simulink model "testemplanner_cs"  (R2023a)
settings: Solver=ode5  StartTime=0.0  StopTime=60  FixedStep=1/1000  RelTol=1e-3
PreLoadFcn:
  | mbxruntime.callbacks.PreLoadFcn(bdroot);
PostLoadFcn:
  | mbxruntime.callbacks.PostLoadFcn(bdroot);
InitFcn:
  | mbxruntime.callbacks.InitFcn(bdroot);
StartFcn:
  | mbxruntime.callbacks.StartFcn(bdroot);
StopFcn:
  | mbxruntime.callbacks.StopFcn(bdroot);
model workspace (MAT data in the model file):
  mbox_table : object (value not decoded)
  model_closed = 0
  sim_status = 0
undefined symbols (not defined in the file): aubr, c_factor, cf, cr, DiscIntNeverNeededParam, global_path_x, global_path_y, KD_PID_distance, KD_PID_speed, KI_PID_distance, KI_PID_speed, KP_PID_distance, KP_PID_speed, la, lb, LQR_K1, LQR_K2, LQR_K3, LQR_K4, m, rack_displacement, right_wheel_ground, tablebr, vubr, vx_break_point
libraries: PreScanSimulinkLibrary x14, Solver_SF x1
(part 5 of 8)

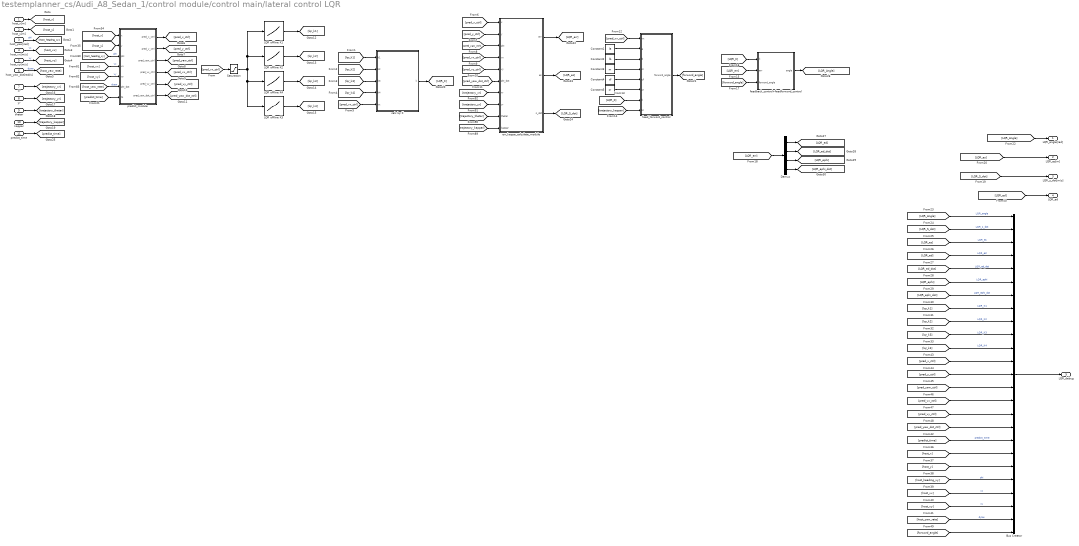
== system testemplanner_cs/Audi_A8_Sedan_1/control module/control main/lateral control LQR ==
  host_x[m] : Inport
  host_y[m] : Inport  Port=2
  host_yaw[rad] : Inport  Port=3
  host_vx[m/s] : Inport  Port=4
  host_vy[m/s] : Inport  Port=5
  host_yaw_dot[rad/s] : Inport  Port=6
  xr : Inport  Port=7
  yr : Inport  Port=8
  thetar : Inport  Port=9
  kappar : Inport  Port=10
  predict_time : Inport  Port=11
  Bus Creator : BusCreator  Inputs=25
  Constant1 : Constant  Value=la
  Constant2 : Constant  Value=lb
  Constant3 : Constant  Value=m
  Constant4 : Constant  Value=cf
  Constant5 : Constant  Value=cr
  Demux : Demux
  LQR offline K1 : Lookup_n-D  NumberOfTableDimensions=1  BreakpointsForDimension1=vx_break_point  Table=LQR_K1  InternalRulePriority=Speed  RndMeth=Simplest
  LQR offline K2 : Lookup_n-D  NumberOfTableDimensions=1  BreakpointsForDimension1=vx_break_point  Table=LQR_K2  InternalRulePriority=Speed  RndMeth=Simplest
  LQR offline K3 : Lookup_n-D  NumberOfTableDimensions=1  BreakpointsForDimension1=vx_break_point  Table=LQR_K3  InternalRulePriority=Speed  RndMeth=Simplest
  LQR offline K4 : Lookup_n-D  NumberOfTableDimensions=1  BreakpointsForDimension1=vx_break_point  Table=LQR_K4  InternalRulePriority=Speed  RndMeth=Simplest
  Saturation : Saturate  UpperLimit=50  LowerLimit=0
  calc lqr K : MATLAB Function  TreatAsAtomicUnit=on
  err_kappa_calculate_module : MATLAB Function  TreatAsAtomicUnit=on
  feed_forword_control : MATLAB Function  TreatAsAtomicUnit=on
  feedback_control+feedforword_control : MATLAB Function  TreatAsAtomicUnit=on
  predict_module : MATLAB Function  TreatAsAtomicUnit=on
  LQR_angle[rad] : Outport  VectorParamsAs1DForOutWhenUnconnected=off
  LQR_es[m] : Outport  Port=2  VectorParamsAs1DForOutWhenUnconnected=off
  LQR_s_dot[m/s] : Outport  Port=3  VectorParamsAs1DForOutWhenUnconnected=off
  LQR_ed : Outport  Port=4  VectorParamsAs1DForOutWhenUnconnected=off
  LQR_debug : Outport  Port=5  VectorParamsAs1DForOutWhenUnconnected=off
  wires:
  [host_vy] -> predict_module/5(vy)  "vy"
  [host_x] -> predict_module/1(x)
  [host_yaw_rate] -> predict_module/6(phi_dot)  "dyaw"
  [host_vx] -> predict_module/4(vx)  "vx"
  [host_y] -> predict_module/2(y)
  [host_heading_xy] -> predict_module/3(phi)  "phi"
  [predict_time] -> predict_module/7(ts)
  host_x[m]/1 -> [host_x]
  host_y[m]/1 -> [host_y]
  host_yaw[rad]/1 -> [host_heading_xy]  "phi"
  host_vx[m/s]/1 -> [host_vx]  "vx"
  host_vy[m/s]/1 -> [host_vy]  "vy"
  host_yaw_dot[rad/s]/1 -> [host_yaw_rate]  "dyaw"
  predict_module/1(pred_x_ctrl) -> [pred_x_ctrl]
  predict_module/2(pred_y_ctrl) -> [pred_y_ctrl]
  predict_module/3(pred_yaw_ctrl) -> [pred_yaw_ctrl]
  predict_module/4(pred_vx_ctrl) -> [pred_vx_ctrl]
  predict_module/5(pred_vy_ctrl) -> [pred_vy_ctrl]
  predict_module/6(pred_yaw_dot_ctrl) -> [pred_yaw_dot_ctrl]
  [pred_vx_ctrl] -> Saturation/1
  LQR offline K1/1 -> [lqr_k1]
  LQR offline K2/1 -> [lqr_k2]
  LQR offline K4/1 -> [lqr_k3]
  LQR offline K3/1 -> [lqr_k4]
  [pred_vx_ctrl] -> calc lqr K/5(vx)
  [lqr_k4] -> calc lqr K/4(k4)
  [lqr_k3] -> calc lqr K/3(k3)
  [lqr_k2] -> calc lqr K/2(k2)
  [lqr_k1] -> calc lqr K/1(k1)
  [pred_x_ctrl] -> err_kappa_calculate_module/1(x)
  [pred_y_ctrl] -> err_kappa_calculate_module/2(y)
  [pred_yaw_ctrl] -> err_kappa_calculate_module/3(phi)
  [pred_vx_ctrl] -> err_kappa_calculate_module/4(vx)
  [pred_vy_ctrl] -> err_kappa_calculate_module/5(vy)
  [pred_yaw_dot_ctrl] -> err_kappa_calculate_module/6(phi_dot)
  xr/1 -> [trajectory_xr]
  yr/1 -> [trajectory_yr]
  thetar/1 -> [trajectory_thetar]
  kappar/1 -> [trajectory_kappar]
  [trajectory_xr] -> err_kappa_calculate_module/7(xr)
  [trajectory_yr] -> err_kappa_calculate_module/8(yr)
  [trajectory_kappar] -> err_kappa_calculate_module/10(kappar)
  [trajectory_thetar] -> err_kappa_calculate_module/9(thetar)
  [pred_vx_ctrl] -> feed_forword_control/1(vx)
  Constant1/1 -> feed_forword_control/2(a)
  Constant2/1 -> feed_forword_control/3(b)
  Constant3/1 -> feed_forword_control/4(m)
  Constant4/1 -> feed_forword_control/5(cf)
  Constant5/1 -> feed_forword_control/6(cr)
  calc lqr K/1(k) -> [LQR_K]
  [LQR_K] -> feed_forword_control/7(k)
  [trajectory_kappar] -> feed_forword_control/8(kr)
  feed_forword_control/1(forword_angle) -> [forword_angle]
  err_kappa_calculate_module/1(err) -> [LQR_err]
  [LQR_err] -> feedback_control+feedforword_control/2(err)
  [LQR_K] -> feedback_control+feedforword_control/1(k)
  [forword_angle] -> feedback_control+feedforword_control/3(forword_angle)
  [LQR_err] -> Demux/1
  err_kappa_calculate_module/2(es) -> [LQR_es]
  err_kappa_calculate_module/3(s_dot) -> [LQR_S_dot]
  [LQR_S_dot] -> LQR_s_dot[m/s]/1
  [LQR_es] -> LQR_es[m]/1
  Saturation/1 -> LQR offline K3/1, LQR offline K4/1, LQR offline K2/1, LQR offline K1/1
  predict_time/1 -> [predict_time]
  Bus Creator/1 -> LQR_debug/1
  feedback_control+feedforword_control/1(angle) -> [LQR_Angle]
  [LQR_Angle] -> LQR_angle[rad]/1
  [LQR_Angle] -> Bus Creator/1  "LQR_angle"
  [LQR_S_dot] -> Bus Creator/2  "LQR_s_dot"
  [LQR_es] -> Bus Creator/3  "LQR_es"
  Demux/1 -> [LQR_ed]
  Demux/2 -> [LQR_ed_dot]
  Demux/3 -> [LQR_ephi]
  Demux/4 -> [LQR_ephi_dot]
  [LQR_ed] -> Bus Creator/4  "LQR_ed"
  [LQR_ed_dot] -> Bus Creator/5  "LQR_ed_dot"
  [LQR_ephi] -> Bus Creator/6  "LQR_ephi"
  [LQR_ephi_dot] -> Bus Creator/7  "LQR_ephi_dot"
  [lqr_k1] -> Bus Creator/8  "LQR_K1"
  [lqr_k2] -> Bus Creator/9  "LQR_K2"
  [lqr_k3] -> Bus Creator/10  "LQR_K3"
  [lqr_k4] -> Bus Creator/11  "LQR_K4"
  [pred_x_ctrl] -> Bus Creator/12
  [pred_y_ctrl] -> Bus Creator/13
  [pred_yaw_ctrl] -> Bus Creator/14
  [pred_vx_ctrl] -> Bus Creator/15
  [pred_vy_ctrl] -> Bus Creator/16
  [pred_yaw_dot_ctrl] -> Bus Creator/17
  [predict_time] -> Bus Creator/18  "predict_time"
  [host_x] -> Bus Creator/19
  [host_y] -> Bus Creator/20
  [host_heading_xy] -> Bus Creator/21  "phi"
  [host_vx] -> Bus Creator/22  "vx"
  [host_vy] -> Bus Creator/23  "vy"
  [host_yaw_rate] -> Bus Creator/24  "dyaw"
  [forword_angle] -> Bus Creator/25
  [LQR_ed] -> LQR_ed/1

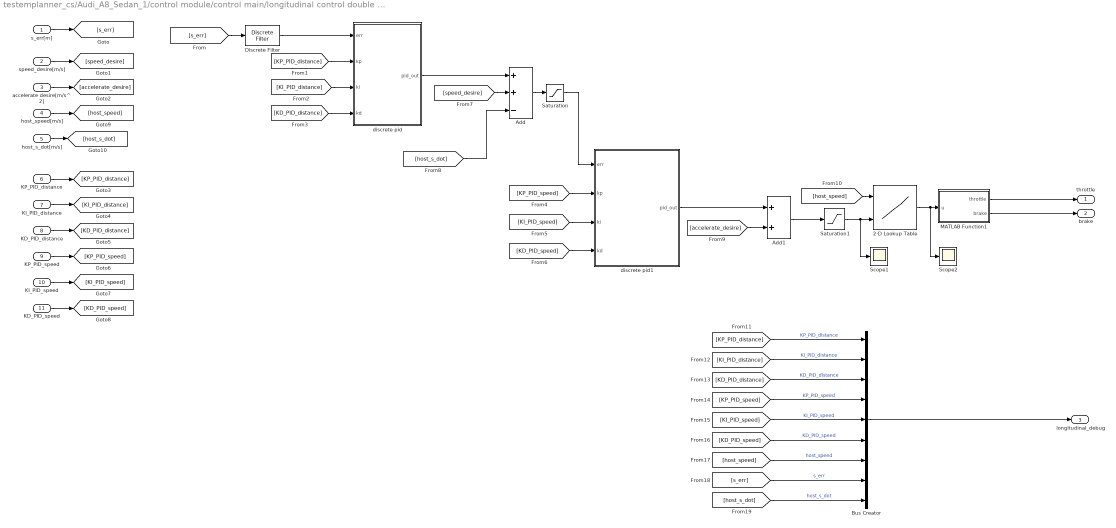
== system testemplanner_cs/Audi_A8_Sedan_1/control module/control main/longitudinal control double PID ==
  s_err[m] : Inport
  speed_desire[m/s] : Inport  Port=2
  accelerate desire[m/s^2] : Inport  Port=3
  host_speed[m/s] : Inport  Port=4
  host_s_dot[m/s] : Inport  Port=5
  KP_PID_distance : Inport  Port=6
  KI_PID_distance : Inport  Port=7
  KD_PID_distance : Inport  Port=8
  KP_PID_speed : Inport  Port=9
  KI_PID_speed : Inport  Port=10
  KD_PID_speed : Inport  Port=11
  2-D Lookup Table : Lookup_n-D  BreakpointsForDimension1=vubr  BreakpointsForDimension2=aubr  Table=tablebr  InternalRulePriority=Speed  RndMeth=Simplest
      settings: InputPortMap=u0,u1
  Add : Sum  Inputs=++-
  Add1 : Sum
  Bus Creator : BusCreator  Inputs=9
  Discrete Filter : DiscreteFilter
  MATLAB Function1 : MATLAB Function  TreatAsAtomicUnit=on
  Saturation : Saturate  UpperLimit=45  LowerLimit=-45
  Saturation1 : Saturate  UpperLimit=5  LowerLimit=-8
  Scope1 : Scope
  Scope2 : Scope
  discrete pid : Subsystem
  discrete pid1 : Subsystem
  throttle : Outport
  brake : Outport  Port=2
  longitudinal_debug : Outport  Port=3
  wires:
  2-D Lookup Table/1 -> Scope2/1, MATLAB Function1/1(u)
  s_err[m]/1 -> [s_err]
  speed_desire[m/s]/1 -> [speed_desire]
  accelerate desire[m/s^2]/1 -> [accelerate_desire]
  KP_PID_distance/1 -> [KP_PID_distance]
  KI_PID_distance/1 -> [KI_PID_distance]
  KD_PID_distance/1 -> [KD_PID_distance]
  KP_PID_speed/1 -> [KP_PID_speed]
  KI_PID_speed/1 -> [KI_PID_speed]
  KD_PID_speed/1 -> [KD_PID_speed]
  [s_err] -> Discrete Filter/1
  [KP_PID_distance] -> discrete pid/2(kp)
  [KI_PID_distance] -> discrete pid/3(ki)
  [KD_PID_distance] -> discrete pid/4(kd)
  [KP_PID_speed] -> discrete pid1/2(kp)
  [KI_PID_speed] -> discrete pid1/3(ki)
  [KD_PID_speed] -> discrete pid1/4(kd)
  host_speed[m/s]/1 -> [host_speed]
  discrete pid/1(pid_out) -> Add/1
  [speed_desire] -> Add/2
  Add/1 -> Saturation/1
  Saturation/1 -> discrete pid1/1(err)
  discrete pid1/1(pid_out) -> Add1/1
  [accelerate_desire] -> Add1/2
  Add1/1 -> Saturation1/1
  Saturation1/1 -> Scope1/1, 2-D Lookup Table/2
  host_s_dot[m/s]/1 -> [host_s_dot]
  [host_s_dot] -> Add/3
  [host_speed] -> 2-D Lookup Table/1
  Discrete Filter/1 -> discrete pid/1(err)
  MATLAB Function1/1(throttle) -> throttle/1
  MATLAB Function1/2(brake) -> brake/1
  [KP_PID_distance] -> Bus Creator/1  "KP_PID_distance"
  [KI_PID_distance] -> Bus Creator/2  "KI_PID_distance"
  [KD_PID_distance] -> Bus Creator/3  "KD_PID_distance"
  [KP_PID_speed] -> Bus Creator/4  "KP_PID_speed"
  [KI_PID_speed] -> Bus Creator/5  "KI_PID_speed"
  [KD_PID_speed] -> Bus Creator/6  "KD_PID_speed"
  [host_speed] -> Bus Creator/7  "host_speed"
  [s_err] -> Bus Creator/8  "s_err"
  [host_s_dot] -> Bus Creator/9  "host_s_dot"
  Bus Creator/1 -> longitudinal_debug/1

== system testemplanner_cs/Audi_A8_Sedan_1/control module/control main/understeer compensate ==
  LQR_angle : Inport
  lateral err : Inport  Port=2
  Add : Sum  Inputs=+-
  Gain : Gain  Gain=0.01
  Manual Switch : ManualSwitch
  LQR_final_angle : Outport
  wires:
  Add/1 -> Manual Switch/2
  Gain/1 -> Add/2
  lateral err/1 -> Gain/1
  LQR_angle/1 -> Add/1, Manual Switch/1
  Manual Switch/1 -> LQR_final_angle/1

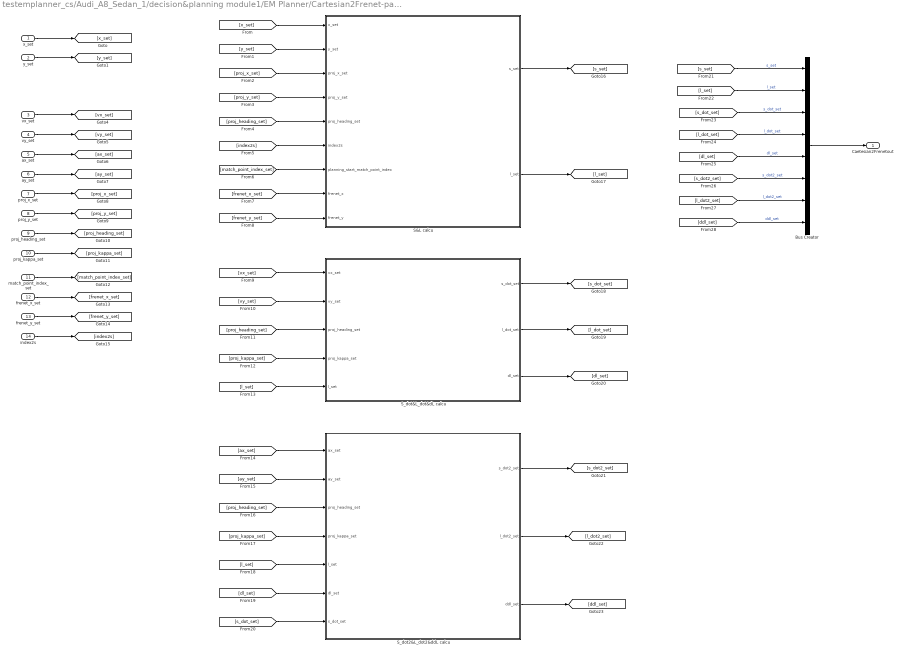
== system testemplanner_cs/Audi_A8_Sedan_1/decision&planning module1/EM Planner/Cartesian2Frenet-panning start point ==
  x_set : Inport
  y_set : Inport  Port=2
  vx_set : Inport  Port=3
  vy_set : Inport  Port=4
  ax_set : Inport  Port=5
  ay_set : Inport  Port=6
  proj_x_set : Inport  Port=7
  proj_y_set : Inport  Port=8
  proj_heading_set : Inport  Port=9
  proj_kappa_set : Inport  Port=10
  match_point_index_set : Inport  Port=11
  frenet_x_set : Inport  Port=12
  frenet_y_set : Inport  Port=13
  index2s : Inport  Port=14
  Bus Creator : BusCreator  Inputs=8
  S&L calcu : MATLAB Function  TreatAsAtomicUnit=on
  "S_dot&L_dot&dL calcu " : MATLAB Function  TreatAsAtomicUnit=on
  S_dot2&L_dot2&ddL calcu : MATLAB Function  TreatAsAtomicUnit=on
  Caetesian2Frenetout : Outport
  wires:
  x_set/1 -> [x_set]
  y_set/1 -> [y_set]
  vx_set/1 -> [vx_set]
  vy_set/1 -> [vy_set]
  ax_set/1 -> [ax_set]
  ay_set/1 -> [ay_set]
  proj_x_set/1 -> [proj_x_set]
  proj_y_set/1 -> [proj_y_set]
  proj_heading_set/1 -> [proj_heading_set]
  proj_kappa_set/1 -> [proj_kappa_set]
  match_point_index_set/1 -> [match_point_index_set]
  frenet_x_set/1 -> [frenet_x_set]
  frenet_y_set/1 -> [frenet_y_set]
  index2s/1 -> [index2s]
  [y_set] -> S&L calcu/2(y_set)
  [proj_x_set] -> S&L calcu/3(proj_x_set)
  [proj_y_set] -> S&L calcu/4(proj_y_set)
  [x_set] -> S&L calcu/1(x_set)
  [proj_heading_set] -> S&L calcu/5(proj_heading_set)
  [index2s] -> S&L calcu/6(index2s)
  [match_point_index_set] -> S&L calcu/7(planning_start_match_point_index)
  [frenet_x_set] -> S&L calcu/8(frenet_x)
  [frenet_y_set] -> S&L calcu/9(frenet_y)
  [vx_set] -> "S_dot&L_dot&dL calcu "/1(vx_set)
  [vy_set] -> "S_dot&L_dot&dL calcu "/2(vy_set)
  [proj_heading_set] -> "S_dot&L_dot&dL calcu "/3(proj_heading_set)
  [proj_kappa_set] -> "S_dot&L_dot&dL calcu "/4(proj_kappa_set)
  S&L calcu/1(s_set) -> [s_set]
  S&L calcu/2(l_set) -> [l_set]
  [l_set] -> "S_dot&L_dot&dL calcu "/5(l_set)
  "S_dot&L_dot&dL calcu "/1(s_dot_set) -> [s_dot_set]
  "S_dot&L_dot&dL calcu "/2(l_dot_set) -> [l_dot_set]
  "S_dot&L_dot&dL calcu "/3(dl_set) -> [dl_set]
  [ax_set] -> S_dot2&L_dot2&ddL calcu/1(ax_set)
  [ay_set] -> S_dot2&L_dot2&ddL calcu/2(ay_set)
  [proj_heading_set] -> S_dot2&L_dot2&ddL calcu/3(proj_heading_set)
  [proj_kappa_set] -> S_dot2&L_dot2&ddL calcu/4(proj_kappa_set)
  [l_set] -> S_dot2&L_dot2&ddL calcu/5(l_set)
  [dl_set] -> S_dot2&L_dot2&ddL calcu/6(dl_set)
  [s_dot_set] -> S_dot2&L_dot2&ddL calcu/7(s_dot_set)
  S_dot2&L_dot2&ddL calcu/1(s_dot2_set) -> [s_dot2_set]
  S_dot2&L_dot2&ddL calcu/2(l_dot2_set) -> [l_dot2_set]
  S_dot2&L_dot2&ddL calcu/3(ddl_set) -> [ddl_set]
  [s_set] -> Bus Creator/1  "s_set"
  [l_set] -> Bus Creator/2  "l_set"
  [s_dot_set] -> Bus Creator/3  "s_dot_set"
  [l_dot_set] -> Bus Creator/4  "l_dot_set"
  [dl_set] -> Bus Creator/5  "dl_set"
  [s_dot2_set] -> Bus Creator/6  "s_dot2_set"
  [l_dot2_set] -> Bus Creator/7  "l_dot2_set"
  [ddl_set] -> Bus Creator/8  "ddl_set"
  Bus Creator/1 -> Caetesian2Frenetout/1

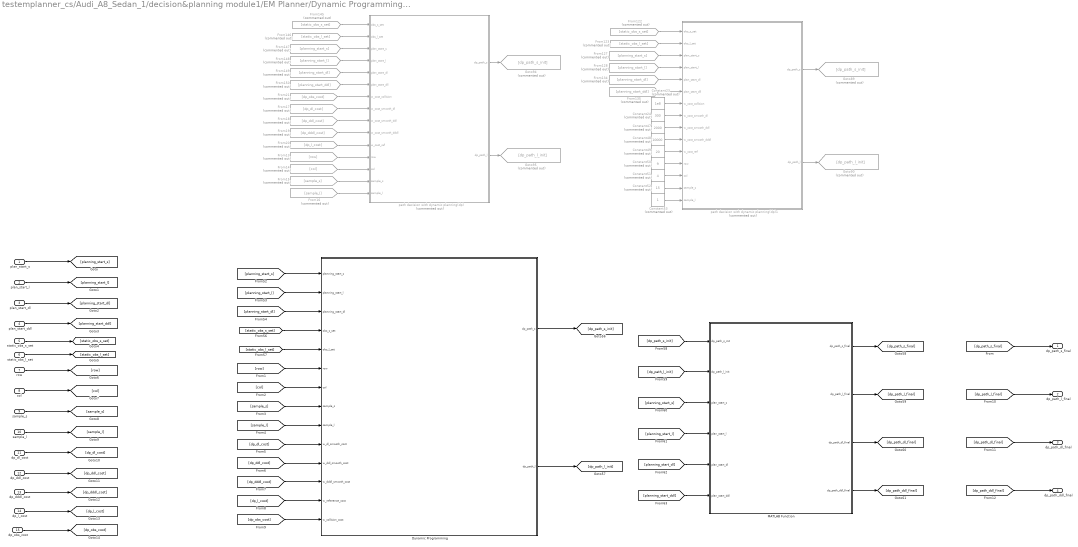
== system testemplanner_cs/Audi_A8_Sedan_1/decision&planning module1/EM Planner/Dynamic Programming&Increase DP Node ==
  plan_start_s : Inport
  plan_start_l : Inport  Port=2
  plan_start_dl : Inport  Port=3
  plan_start_ddl : Inport  Port=4
  static_obs_s_set : Inport  Port=5
  static_obs_l_set : Inport  Port=6
  row : Inport  Port=7
  col : Inport  Port=8
  sample_s : Inport  Port=9
  sample_l : Inport  Port=10
  dp_dl_cost : Inport  Port=11
  dp_ddl_cost : Inport  Port=12
  dp_dddl_cost : Inport  Port=13
  dp_l_cost : Inport  Port=14
  dp_obs_cost : Inport  Port=15
  Constant23 : Constant  Commented=on  Value=1e8
  Constant24 : Constant  Commented=on  Value=300
  Constant47 : Constant  Commented=on  Value=2000
  Constant48 : Constant  Commented=on  Value=10000
  Constant49 : Constant  Commented=on  Value=20
  Constant50 : Constant  Commented=on  Value=9
  Constant51 : Constant  Commented=on  Value=4
  Constant52 : Constant  Commented=on  Value=15
  Constant53 : Constant  Commented=on
  Dynamic Programming : MATLAB Function  TreatAsAtomicUnit=on
  From122 : From  Commented=on  GotoTag=static_obs_s_set
  From123 : From  Commented=on  GotoTag=static_obs_l_set
  From127 : From  Commented=on  GotoTag=planning_start_s
  From128 : From  Commented=on  GotoTag=planning_start_l
  From13 : From  Commented=on  GotoTag=row
  From134 : From  Commented=on  GotoTag=planning_start_dl
  From135 : From  Commented=on  GotoTag=planning_start_ddl
  From14 : From  Commented=on  GotoTag=col
  From145 : From  Commented=on  GotoTag=static_obs_s_set
  From146 : From  Commented=on  GotoTag=static_obs_l_set
  From147 : From  Commented=on  GotoTag=planning_start_s
  From148 : From  Commented=on  GotoTag=planning_start_l
  From149 : From  Commented=on  GotoTag=planning_start_dl
  From15 : From  Commented=on  GotoTag=sample_s
  From150 : From  Commented=on  GotoTag=planning_start_ddl
  From16 : From  Commented=on  GotoTag=sample_l
  From17 : From  Commented=on  GotoTag=dp_dl_cost
  From18 : From  Commented=on  GotoTag=dp_ddl_cost
  From19 : From  Commented=on  GotoTag=dp_dddl_cost
  From20 : From  Commented=on  GotoTag=dp_l_cost
  From21 : From  Commented=on  GotoTag=dp_obs_cost
  Goto89 : Goto  Commented=on  GotoTag=dp_path_s_init
  Goto90 : Goto  Commented=on  GotoTag=dp_path_l_init
  Goto94 : Goto  Commented=on  GotoTag=dp_path_s_init
  Goto95 : Goto  Commented=on  GotoTag=dp_path_l_init
  MATLAB Function : MATLAB Function  TreatAsAtomicUnit=on
  path decision with dynamic planning(dp) : MATLAB Function  Commented=on  TreatAsAtomicUnit=on
  path decision with dynamic planning(dp)1 : MATLAB Function  Commented=on  TreatAsAtomicUnit=on
  dp_path_s_final : Outport
  dp_path_l_final : Outport  Port=2
  dp_path_dl_final : Outport  Port=3
  dp_path_ddl_final : Outport  Port=4
  wires:
  Constant23/1 -> path decision with dynamic planning(dp)1/7(w_cost_collision)
  From21/1 -> path decision with dynamic planning(dp)/7(w_cost_collision)
  Constant47/1 -> path decision with dynamic planning(dp)1/9(w_cost_smooth_ddl)
  Constant49/1 -> path decision with dynamic planning(dp)1/11(w_cost_ref)
  Constant24/1 -> path decision with dynamic planning(dp)1/8(w_cost_smooth_dl)
  [row] -> Dynamic Programming/6(row)
  [sample_s] -> Dynamic Programming/8(sample_s)
  From19/1 -> path decision with dynamic planning(dp)/10(w_cost_smooth_dddl)
  Constant50/1 -> path decision with dynamic planning(dp)1/12(row)
  MATLAB Function/3(dp_path_dl_final) -> [dp_path_dl_final]
  [col] -> Dynamic Programming/7(col)
  MATLAB Function/1(dp_path_s_final) -> [dp_path_s_final]
  Constant48/1 -> path decision with dynamic planning(dp)1/10(w_cost_smooth_dddl)
  From128/1 -> path decision with dynamic planning(dp)1/4(plan_start_l)
  From123/1 -> path decision with dynamic planning(dp)1/2(obs_l_set)
  From134/1 -> path decision with dynamic planning(dp)1/5(plan_start_dl)
  path decision with dynamic planning(dp)/2(dp_path_l) -> Goto95/1
  path decision with dynamic planning(dp)1/1(dp_path_s) -> Goto89/1
  [planning_start_l] -> MATLAB Function/4(plan_start_l)
  [planning_start_dl] -> Dynamic Programming/3(planning_start_dl)
  From17/1 -> path decision with dynamic planning(dp)/8(w_cost_smooth_dl)
  From16/1 -> path decision with dynamic planning(dp)/15(sample_l)
  path decision with dynamic planning(dp)1/2(dp_path_l) -> Goto90/1
  Constant52/1 -> path decision with dynamic planning(dp)1/14(sample_s)
  Constant51/1 -> path decision with dynamic planning(dp)1/13(col)
  From135/1 -> path decision with dynamic planning(dp)1/6(plan_start_dll)
  From149/1 -> path decision with dynamic planning(dp)/5(plan_start_dl)
  From18/1 -> path decision with dynamic planning(dp)/9(w_cost_smooth_ddl)
  From122/1 -> path decision with dynamic planning(dp)1/1(obs_s_set)
  [dp_ddl_cost] -> Dynamic Programming/11(w_ddl_smooth_cost)
  Constant53/1 -> path decision with dynamic planning(dp)1/15(sample_l)
  [planning_start_l] -> Dynamic Programming/2(planning_start_l)
  From127/1 -> path decision with dynamic planning(dp)1/3(plan_start_s)
  [planning_start_s] -> MATLAB Function/3(plan_start_s)
  Dynamic Programming/1(dp_path_s) -> [dp_path_s_init]
  [dp_l_cost] -> Dynamic Programming/13(w_reference_cost)
  [static_obs_l_set] -> Dynamic Programming/5(obs_l_set)
  From15/1 -> path decision with dynamic planning(dp)/14(sample_s)
  From13/1 -> path decision with dynamic planning(dp)/12(row)
  [planning_start_s] -> Dynamic Programming/1(planning_start_s)
  From146/1 -> path decision with dynamic planning(dp)/2(obs_l_set)
  [dp_path_s_init] -> MATLAB Function/1(dp_path_s_init)
  [planning_start_ddl] -> MATLAB Function/6(plan_start_ddl)
  [static_obs_s_set] -> Dynamic Programming/4(obs_s_set)
  [dp_obs_cost] -> Dynamic Programming/14(w_collision_cost)
  [planning_start_dl] -> MATLAB Function/5(plan_start_dl)
  Dynamic Programming/2(dp_path_l) -> [dp_path_l_init]
  MATLAB Function/4(dp_path_ddl_final) -> [dp_path_ddl_final]
  [dp_path_l_init] -> MATLAB Function/2(dp_path_l_init)
  [dp_dl_cost] -> Dynamic Programming/10(w_dl_smooth_cost)
  [sample_l] -> Dynamic Programming/9(sample_l)
  MATLAB Function/2(dp_path_l_final) -> [dp_path_l_final]
  From14/1 -> path decision with dynamic planning(dp)/13(col)
  From145/1 -> path decision with dynamic planning(dp)/1(obs_s_set)
  path decision with dynamic planning(dp)/1(dp_path_s) -> Goto94/1
  From20/1 -> path decision with dynamic planning(dp)/11(w_cost_ref)
  From150/1 -> path decision with dynamic planning(dp)/6(plan_start_dll)
  From147/1 -> path decision with dynamic planning(dp)/3(plan_start_s)
  [dp_dddl_cost] -> Dynamic Programming/12(w_dddl_smooth_cost)
  From148/1 -> path decision with dynamic planning(dp)/4(plan_start_l)
  plan_start_s/1 -> [planning_start_s]
  plan_start_l/1 -> [planning_start_l]
  plan_start_dl/1 -> [planning_start_dl]
  plan_start_ddl/1 -> [planning_start_ddl]
  static_obs_s_set/1 -> [static_obs_s_set]
  static_obs_l_set/1 -> [static_obs_l_set]
  row/1 -> [row]
  col/1 -> [col]
  sample_s/1 -> [sample_s]
  sample_l/1 -> [sample_l]
  dp_dl_cost/1 -> [dp_dl_cost]
  dp_ddl_cost/1 -> [dp_ddl_cost]
  dp_dddl_cost/1 -> [dp_dddl_cost]
  dp_l_cost/1 -> [dp_l_cost]
  dp_obs_cost/1 -> [dp_obs_cost]
  [dp_path_s_final] -> dp_path_s_final/1
  [dp_path_l_final] -> dp_path_l_final/1
  [dp_path_dl_final] -> dp_path_dl_final/1
  [dp_path_ddl_final] -> dp_path_ddl_final/1

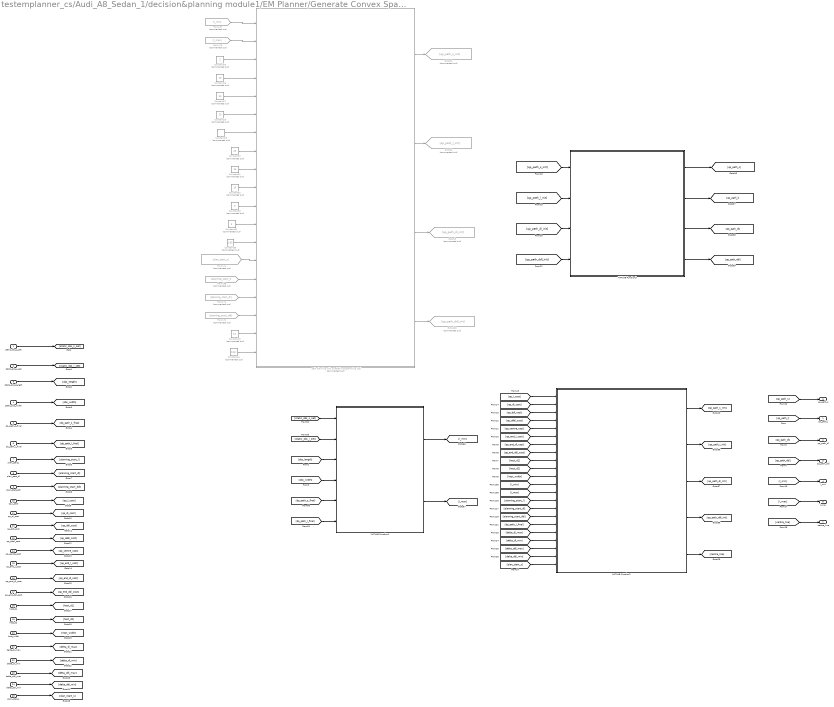
== system testemplanner_cs/Audi_A8_Sedan_1/decision&planning module1/EM Planner/Generate Convex Space&Quadratic Programming ==
  static_obs_s_set : Inport
  static_obs_l_set : Inport  Port=2
  static_obs_length : Inport  Port=3
  static_obs_width : Inport  Port=4
  dp_path_s_final : Inport  Port=5
  dp_path_l_final : Inport  Port=6
  plan_start_l : Inport  Port=7
  plan_start_dl : Inport  Port=8
  plan_start_ddl : Inport  Port=9
  qp_l_cost : Inport  Port=10
  qp_dl_cost : Inport  Port=11
  qp_ddl_cost : Inport  Port=12
  qp_dddl_cost : Inport  Port=13
  qp_centre_cost : Inport  Port=14
  qp_end_l_cost : Inport  Port=15
  qp_end_dl_cost : Inport  Port=16
  qp_end_ddl_cost : Inport  Port=17
  host_d1 : Inport  Port=18
  host_d2 : Inport  Port=19
  host_width : Inport  Port=20
  delta_dl_max : Inport  Port=21
  delta_dl_min : Inport  Port=22
  delta_ddl_max : Inport  Port=23
  delta_ddl_min : Inport  Port=24
  plan_start_s : Inport  Port=25
  Constant25 : Constant  Commented=on  Value=2
  Constant{26,30..32} (4 alike) : Constant  Commented=on  Value=15
  Constant27 : Constant  Commented=on  Value=50
  Constant28 : Constant  Commented=on  Value=20
  Constant29 : Constant  Commented=on  Value=25000
  Constant33 : Constant  Commented=on  Value=3
  Constant34 : Constant  Commented=on  Value=3
  Constant35 : Constant  Commented=on  Value=1.63
  Constant45 : Constant  Commented=on  Value=0.1
  Constant46 : Constant  Commented=on  Value=0.02
  From137 : From  Commented=on  GotoTag=l_min
  From138 : From  Commented=on  GotoTag=planning_start_l
  From170 : From  Commented=on  GotoTag=l_max
  From171 : From  Commented=on  GotoTag=planning_start_dl
  From172 : From  Commented=on  GotoTag=planning_start_ddl
  From174 : From  Commented=on  GotoTag=plan_start_s
  Goto100 : Goto  Commented=on  GotoTag=qp_path_ddl_init
  Goto91 : Goto  Commented=on  GotoTag=qp_path_s_init
  Goto92 : Goto  Commented=on  GotoTag=qp_path_l_init
  Goto93 : Goto  Commented=on  GotoTag=qp_path_dl_init
  MATLAB Function1 : MATLAB Function  TreatAsAtomicUnit=on
  MATLAB Function2 : MATLAB Function  TreatAsAtomicUnit=on
  MATLAB Function3 : MATLAB Function  TreatAsAtomicUnit=on
  path planning with quadratic programming (qp) : MATLAB Function  Commented=on  TreatAsAtomicUnit=on
  qp_path_l : Outport
  qp_path_dl : Outport  Port=2
  qp_path_ddl : Outport  Port=3
  l_min : Outport  Port=4
  l_max : Outport  Port=5
  qp_path_s : Outport  Port=6
  centre_line : Outport  Port=7
  wires:
  From170/1 -> path planning with quadratic programming (qp)/2(l_max)
  path planning with quadratic programming (qp)/2(qp_path_l) -> Goto92/1
  [qp_path_ddl_init] -> MATLAB Function3/4(qp_path_ddl)
  path planning with quadratic programming (qp)/1(qp_path_s) -> Goto91/1
  [qp_end_l_cost] -> MATLAB Function2/6(w_end_l_cost)
  MATLAB Function2/3(qp_path_dl) -> [qp_path_dl_init]
  Constant35/1 -> path planning with quadratic programming (qp)/13(host_w)
  Constant26/1 -> path planning with quadratic programming (qp)/4(w_cost_dl)
  MATLAB Function3/2(qp_path_l_final) -> [qp_path_l]
  Constant27/1 -> path planning with quadratic programming (qp)/5(w_cost_ddl)
  [static_obs_s_set] -> MATLAB Function1/1(static_obs_s_set)
  Constant34/1 -> path planning with quadratic programming (qp)/12(host_d2)
  MATLAB Function2/2(qp_path_l) -> [qp_path_l_init]
  MATLAB Function3/1(qp_path_s_final) -> [qp_path_s]
  Constant33/1 -> path planning with quadratic programming (qp)/11(host_d1)
  [qp_path_dl_init] -> MATLAB Function3/3(qp_path_dl)
  Constant29/1 -> path planning with quadratic programming (qp)/7(w_cost_centre)
  [l_min] -> MATLAB Function2/12(lmin)
  Constant25/1 -> path planning with quadratic programming (qp)/3(w_cost_l)
  Constant28/1 -> path planning with quadratic programming (qp)/6(w_cost_dddl)
  From172/1 -> path planning with quadratic programming (qp)/17(plan_start_ddl)
  From138/1 -> path planning with quadratic programming (qp)/15(plan_start_l)
  From137/1 -> path planning with quadratic programming (qp)/1(l_min)
  [static_obs_l_set] -> MATLAB Function1/2(static_obs_l_set)
  [dp_path_l_final] -> MATLAB Function2/17(dp_path_l_final)
  path planning with quadratic programming (qp)/4(qp_path_ddl) -> Goto100/1
  [qp_end_dl_cost] -> MATLAB Function2/7(w_end_dl_cost)
  MATLAB Function3/4(qp_path_ddl_final) -> [qp_path_ddl]
  [host_d1] -> MATLAB Function2/9(d1)
  path planning with quadratic programming (qp)/3(qp_path_dl) -> Goto93/1
  [qp_l_cost] -> MATLAB Function2/1(w_ref_cost)
  Constant45/1 -> path planning with quadratic programming (qp)/18(delta_dl_max)
  From174/1 -> path planning with quadratic programming (qp)/14(plan_start_s)
  [planning_start_dl] -> MATLAB Function2/15(plan_start_dl)
  From171/1 -> path planning with quadratic programming (qp)/16(plan_start_dl)
  Constant30/1 -> path planning with quadratic programming (qp)/8(w_cost_end_l)
  [qp_ddl_cost] -> MATLAB Function2/3(w_ddl_cost)
  [obs_width] -> MATLAB Function1/4(obs_width)
  [obs_length] -> MATLAB Function1/3(obs_length)
  [planning_start_ddl] -> MATLAB Function2/16(plan_start_ddl)
  [l_max] -> MATLAB Function2/13(lmax)
  [host_width] -> MATLAB Function2/11(width)
  [qp_path_l_init] -> MATLAB Function3/2(qp_path_l)
  [qp_centre_cost] -> MATLAB Function2/5(w_centre_cost)
  [qp_dl_cost] -> MATLAB Function2/2(w_dl_cost)
  [dp_path_s_final] -> MATLAB Function1/5(dp_path_s)
  [qp_dddl_cost] -> MATLAB Function2/4(w_dddl_cost)
  [planning_start_l] -> MATLAB Function2/14(plan_start_l)
  Constant31/1 -> path planning with quadratic programming (qp)/9(w_cost_end_dl)
  [host_d2] -> MATLAB Function2/10(d2)
  Constant32/1 -> path planning with quadratic programming (qp)/10(w_cost_end_ddl)
  MATLAB Function2/4(qp_path_ddl) -> [qp_path_ddl_init]
  [qp_end_ddl_cost] -> MATLAB Function2/8(w_end_ddl_cost)
  MATLAB Function1/2(l_max) -> [l_max]
  [dp_path_l_final] -> MATLAB Function1/6(dp_path_l)
  MATLAB Function1/1(l_min) -> [l_min]
  MATLAB Function3/3(qp_path_dl_final) -> [qp_path_dl]
  Constant46/1 -> path planning with quadratic programming (qp)/19(delta_ddl_max)
  [qp_path_s_init] -> MATLAB Function3/1(qp_path_s)
  static_obs_s_set/1 -> [static_obs_s_set]
  static_obs_l_set/1 -> [static_obs_l_set]
  static_obs_length/1 -> [obs_length]
  static_obs_width/1 -> [obs_width]
  dp_path_s_final/1 -> [dp_path_s_final]
  dp_path_l_final/1 -> [dp_path_l_final]
  plan_start_l/1 -> [planning_start_l]
  plan_start_dl/1 -> [planning_start_dl]
  plan_start_ddl/1 -> [planning_start_ddl]
  [qp_path_l] -> qp_path_l/1
  [qp_path_dl] -> qp_path_dl/1
  [qp_path_ddl] -> qp_path_ddl/1
  qp_l_cost/1 -> [qp_l_cost]
  qp_dl_cost/1 -> [qp_dl_cost]
  qp_ddl_cost/1 -> [qp_ddl_cost]
  qp_dddl_cost/1 -> [qp_dddl_cost]
  qp_centre_cost/1 -> [qp_centre_cost]
  qp_end_l_cost/1 -> [qp_end_l_cost]
  qp_end_dl_cost/1 -> [qp_end_dl_cost]
  qp_end_ddl_cost/1 -> [qp_end_ddl_cost]
  host_d1/1 -> [host_d1]
  host_d2/1 -> [host_d2]
  host_width/1 -> [host_width]
  [l_min] -> l_min/1
  [l_max] -> l_max/1
  [qp_path_s] -> qp_path_s/1
  MATLAB Function2/1(qp_path_s) -> [qp_path_s_init]
  [delta_dl_max] -> MATLAB Function2/18(delta_dl_max)
  [delta_dl_min] -> MATLAB Function2/19(delta_dl_min)
  [delta_ddl_max] -> MATLAB Function2/20(delta_ddl_max)
  [delta_ddl_min] -> MATLAB Function2/21(delta_ddl_min)
  [plan_start_s] -> MATLAB Function2/22(plan_start_s)
  delta_dl_max/1 -> [delta_dl_max]
  delta_dl_min/1 -> [delta_dl_min]
  delta_ddl_max/1 -> [delta_ddl_max]
  delta_ddl_min/1 -> [delta_ddl_min]
  plan_start_s/1 -> [plan_start_s]
  MATLAB Function2/5(centre_line) -> [centre_line]
  [centre_line] -> centre_line/1

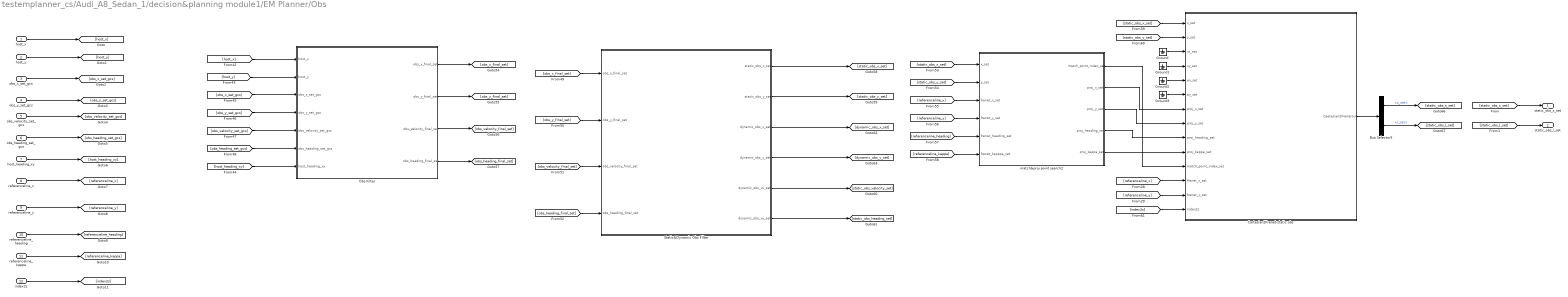
== system testemplanner_cs/Audi_A8_Sedan_1/decision&planning module1/EM Planner/Obs ==
  host_x : Inport
  host_y : Inport  Port=2
  obs_x_set_gcs : Inport  Port=3
  obs_y_set_gcs : Inport  Port=4
  obs_velocity_set_gcs : Inport  Port=5
  obs_heading_set_gcs : Inport  Port=6
  host_heading_xy : Inport  Port=7
  referenceline_x : Inport  Port=8
  referenceline_y : Inport  Port=9
  referenceline_heading : Inport  Port=10
  referenceline_kappa : Inport  Port=11
  index2s : Inport  Port=12
  Bus Selector5 : BusSelector  OutputSignals=s_set,l_set
  Cartesian2Frenet-static obs : Subsystem
  Ground{,1..3} (4 alike) : Ground
  Obs Filter : MATLAB Function  TreatAsAtomicUnit=on
  Static&Dynamic Obs Filter : MATLAB Function  TreatAsAtomicUnit=on
  match&proj point search2 : MATLAB Function  TreatAsAtomicUnit=on
  static_obs_s_set : Outport
  static_obs_l_set : Outport  Port=2
  wires:
  [referenceline_kappa] -> match&proj point search2/6(frenet_kapppa_set)
  Bus Selector5/1 -> [static_obs_s_set]  "<s_set>"
  [host_x] -> Obs Filter/1(host_x)
  Static&Dynamic Obs Filter/6(dynamic_obs_vy_set) -> [static_obs_heading_set]
  match&proj point search2/2(proj_x_set) -> Cartesian2Frenet-static obs/7(proj_x_set)
  Obs Filter/2(obs_y_final_set) -> [obs_y_final_set]
  Static&Dynamic Obs Filter/2(static_obs_y_set) -> [static_obs_y_set]
  Obs Filter/3(obs_velocity_final_set) -> [obs_velocity_final_set]
  Static&Dynamic Obs Filter/1(static_obs_x_set) -> [static_obs_x_set]
  [referenceline_x] -> match&proj point search2/3(frenet_x_set)
  [referenceline_y] -> Cartesian2Frenet-static obs/13(frenet_y_set)
  Bus Selector5/2 -> [static_obs_l_set]  "<l_set>"
  [obs_y_final_set] -> Static&Dynamic Obs Filter/2(obs_y_final_set)
  [host_y] -> Obs Filter/2(host_y)
  [referenceline_x] -> Cartesian2Frenet-static obs/12(frenet_x_set)
  Obs Filter/1(obs_x_final_set) -> [obs_x_final_set]
  Ground2/1 -> Cartesian2Frenet-static obs/5(ax_set)
  Static&Dynamic Obs Filter/4(dynamic_obs_y_set) -> [dynamic_obs_y_set]
  [obs_heading_final_set] -> Static&Dynamic Obs Filter/4(obs_heading_final_set)
  [obs_velocity_final_set] -> Static&Dynamic Obs Filter/3(obs_velocity_final_set)
  [obs_x_set_gcs] -> Obs Filter/3(obs_x_set_gcs)
  Ground/1 -> Cartesian2Frenet-static obs/3(vx_set)
  Obs Filter/4(obs_heading_final_set) -> [obs_heading_final_set]
  match&proj point search2/4(proj_heading_set) -> Cartesian2Frenet-static obs/9(proj_heading_set)
  Static&Dynamic Obs Filter/5(dynamic_obs_vx_set) -> [static_obs_velocity_set]
  [static_obs_x_set] -> Cartesian2Frenet-static obs/1(x_set)
  [obs_x_final_set] -> Static&Dynamic Obs Filter/1(obs_x_final_set)
  [obs_y_set_gcs] -> Obs Filter/4(obs_y_set_gcs)
  [obs_heading_set_gcs] -> Obs Filter/6(obs_heading_set_gcs)
  Ground1/1 -> Cartesian2Frenet-static obs/4(vy_set)
  [index2s] -> Cartesian2Frenet-static obs/14(index2s)
  [host_heading_xy] -> Obs Filter/7(host_heading_xy)
  [referenceline_y] -> match&proj point search2/4(frenet_y_set)
  Static&Dynamic Obs Filter/3(dynamic_obs_x_set) -> [dynamic_obs_x_set]
  match&proj point search2/1(match_point_index_set) -> Cartesian2Frenet-static obs/11(match_point_index_set)
  [static_obs_y_set] -> Cartesian2Frenet-static obs/2(y_set)
  Cartesian2Frenet-static obs/1(Caetesian2Frenetout) -> Bus Selector5/1
  [referenceline_heading] -> match&proj point search2/5(frenet_heading_set)
  match&proj point search2/5(proj_kappa_set) -> Cartesian2Frenet-static obs/10(proj_kappa_set)
  [obs_velocity_set_gcs] -> Obs Filter/5(obs_velocity_set_gcs)
  [static_obs_x_set] -> match&proj point search2/1(x_set)
  Ground3/1 -> Cartesian2Frenet-static obs/6(ay_set)
  match&proj point search2/3(proj_y_set) -> Cartesian2Frenet-static obs/8(proj_y_set)
  [static_obs_y_set] -> match&proj point search2/2(y_set)
  host_x/1 -> [host_x]
  host_y/1 -> [host_y]
  obs_x_set_gcs/1 -> [obs_x_set_gcs]
  obs_y_set_gcs/1 -> [obs_y_set_gcs]
  obs_velocity_set_gcs/1 -> [obs_velocity_set_gcs]
  obs_heading_set_gcs/1 -> [obs_heading_set_gcs]
  host_heading_xy/1 -> [host_heading_xy]
  referenceline_x/1 -> [referenceline_x]
  referenceline_y/1 -> [referenceline_y]
  referenceline_heading/1 -> [referenceline_heading]
  referenceline_kappa/1 -> [referenceline_kappa]
  index2s/1 -> [index2s]
  [static_obs_s_set] -> static_obs_s_set/1
  [static_obs_l_set] -> static_obs_l_set/1

== system testemplanner_cs/Box_1/SELF_Demux/compas converter/cart2compas ==
  Angle [deg] : Inport
  Constant : Constant  Value=90
  Constant1 : Constant  Value=360
  Gain : Gain  Gain=1/360
  Gain1 : Gain  Gain=360
  Gain2 : Gain  Gain=-1
  Rounding Function : Rounding
  Sum : Sum  Inputs=|-+
  Sum1 : Sum  Inputs=-+|
  Sum2 : Sum  Inputs=++|
  heading [deg] : Outport
  wires:
  Gain/1 -> Rounding Function/1
  Rounding Function/1 -> Gain1/1
  Gain1/1 -> Sum/1
  Angle [deg]/1 -> Sum1/2
  Sum/1 -> Gain2/1
  Sum1/1 -> Gain/1, Sum/2
  Constant/1 -> Sum1/1
  Gain2/1 -> Sum2/2
  Constant1/1 -> Sum2/1
  Sum2/1 -> heading [deg]/1

== system testemplanner_cs/Box_2/SELF_Demux/compas converter/cart2compas ==
  Angle [deg] : Inport
  Constant : Constant  Value=90
  Constant1 : Constant  Value=360
  Gain : Gain  Gain=1/360
  Gain1 : Gain  Gain=360
  Gain2 : Gain  Gain=-1
  Rounding Function : Rounding
  Sum : Sum  Inputs=|-+
  Sum1 : Sum  Inputs=-+|
  Sum2 : Sum  Inputs=++|
  heading [deg] : Outport
  wires:
  Gain/1 -> Rounding Function/1
  Rounding Function/1 -> Gain1/1
  Gain1/1 -> Sum/1
  Angle [deg]/1 -> Sum1/2
  Sum/1 -> Gain2/1
  Sum1/1 -> Gain/1, Sum/2
  Constant/1 -> Sum1/1
  Gain2/1 -> Sum2/2
  Constant1/1 -> Sum2/1
  Sum2/1 -> heading [deg]/1

== system testemplanner_cs/Box_3/SELF_Demux/compas converter/cart2compas ==
  Angle [deg] : Inport
  Constant : Constant  Value=90
  Constant1 : Constant  Value=360
  Gain : Gain  Gain=1/360
  Gain1 : Gain  Gain=360
  Gain2 : Gain  Gain=-1
  Rounding Function : Rounding
  Sum : Sum  Inputs=|-+
  Sum1 : Sum  Inputs=-+|
  Sum2 : Sum  Inputs=++|
  heading [deg] : Outport
  wires:
  Gain/1 -> Rounding Function/1
  Rounding Function/1 -> Gain1/1
  Gain1/1 -> Sum/1
  Angle [deg]/1 -> Sum1/2
  Sum/1 -> Gain2/1
  Sum1/1 -> Gain/1, Sum/2
  Constant/1 -> Sum1/1
  Gain2/1 -> Sum2/2
  Constant1/1 -> Sum2/1
  Sum2/1 -> heading [deg]/1

== system testemplanner_cs/Box_4/SELF_Demux/compas converter/cart2compas ==
  Angle [deg] : Inport
  Constant : Constant  Value=90
  Constant1 : Constant  Value=360
  Gain : Gain  Gain=1/360
  Gain1 : Gain  Gain=360
  Gain2 : Gain  Gain=-1
  Rounding Function : Rounding
  Sum : Sum  Inputs=|-+
  Sum1 : Sum  Inputs=-+|
  Sum2 : Sum  Inputs=++|
  heading [deg] : Outport
  wires:
  Gain/1 -> Rounding Function/1
  Rounding Function/1 -> Gain1/1
  Gain1/1 -> Sum/1
  Angle [deg]/1 -> Sum1/2
  Sum/1 -> Gain2/1
  Sum1/1 -> Gain/1, Sum/2
  Constant/1 -> Sum1/1
  Gain2/1 -> Sum2/2
  Constant1/1 -> Sum2/1
  Sum2/1 -> heading [deg]/1

== system testemplanner_cs/Box_5/SELF_Demux/compas converter/cart2compas ==
  Angle [deg] : Inport
  Constant : Constant  Value=90
  Constant1 : Constant  Value=360
  Gain : Gain  Gain=1/360
  Gain1 : Gain  Gain=360
  Gain2 : Gain  Gain=-1
  Rounding Function : Rounding
  Sum : Sum  Inputs=|-+
  Sum1 : Sum  Inputs=-+|
  Sum2 : Sum  Inputs=++|
  heading [deg] : Outport
  wires:
  Gain/1 -> Rounding Function/1
  Rounding Function/1 -> Gain1/1
  Gain1/1 -> Sum/1
  Angle [deg]/1 -> Sum1/2
  Sum/1 -> Gain2/1
  Sum1/1 -> Gain/1, Sum/2
  Constant/1 -> Sum1/1
  Gain2/1 -> Sum2/2
  Constant1/1 -> Sum2/1
  Sum2/1 -> heading [deg]/1

== system testemplanner_cs/Box_6/SELF_Demux/compas converter/cart2compas ==
  Angle [deg] : Inport
  Constant : Constant  Value=90
  Constant1 : Constant  Value=360
  Gain : Gain  Gain=1/360
  Gain1 : Gain  Gain=360
  Gain2 : Gain  Gain=-1
  Rounding Function : Rounding
  Sum : Sum  Inputs=|-+
  Sum1 : Sum  Inputs=-+|
  Sum2 : Sum  Inputs=++|
  heading [deg] : Outport
  wires:
  Gain/1 -> Rounding Function/1
  Rounding Function/1 -> Gain1/1
  Gain1/1 -> Sum/1
  Angle [deg]/1 -> Sum1/2
  Sum/1 -> Gain2/1
  Sum1/1 -> Gain/1, Sum/2
  Constant/1 -> Sum1/1
  Gain2/1 -> Sum2/2
  Constant1/1 -> Sum2/1
  Sum2/1 -> heading [deg]/1

== system testemplanner_cs/Audi_A8_Sedan_1/control module/control main/longitudinal control double PID/discrete pid ==
  err : Inport
  kp : Inport  Port=2
  ki : Inport  Port=3
  kd : Inport  Port=4
  Add2 : Sum  Inputs=+++
  Add3 : Sum
  Add4 : Sum  Inputs=+-
  Delay3 : Delay  DelayLength=1
  Delay4 : Delay  DelayLength=1
  Divide : Product  Inputs=**
  Divide1 : Product  Inputs=**
  Divide2 : Product  Inputs=**
  Gain : Gain  Gain=0.01
  pid_out : Outport
  wires:
  [KD_PID_distance] -> Divide2/2
  err/1 -> Delay4/1, Divide/2, Add3/1, Add4/1
  Divide/1 -> Add2/1
  Divide2/1 -> Add2/3
  Add3/1 -> Gain/1, Divide1/1
  Delay4/1 -> Add4/2
  [KP_PID_distance] -> Divide/1
  Divide1/1 -> Add2/2
  Delay3/1 -> Add3/2
  [KI_PID_distance] -> Divide1/2
  Add4/1 -> Divide2/1
  Add2/1 -> pid_out/1
  kp/1 -> [KP_PID_distance]
  ki/1 -> [KI_PID_distance]
  kd/1 -> [KD_PID_distance]
  Gain/1 -> Delay3/1

== system testemplanner_cs/Audi_A8_Sedan_1/control module/control main/longitudinal control double PID/discrete pid1 ==
  err : Inport
  kp : Inport  Port=2
  ki : Inport  Port=3
  kd : Inport  Port=4
  Add2 : Sum  Inputs=+++
  Add3 : Sum
  Add4 : Sum  Inputs=+-
  Delay3 : Delay  DelayLength=1
  Delay4 : Delay  DelayLength=1
  Divide : Product  Inputs=**
  Divide1 : Product  Inputs=**
  Divide2 : Product  Inputs=**
  Gain : Gain  Gain=0.01
  pid_out : Outport
  wires:
  Gain/1 -> Delay3/1
  kd/1 -> [KD_PID_distance]
  ki/1 -> [KI_PID_distance]
  kp/1 -> [KP_PID_distance]
  Add2/1 -> pid_out/1
  Add4/1 -> Divide2/1
  [KI_PID_distance] -> Divide1/2
  Delay3/1 -> Add3/2
  Divide1/1 -> Add2/2
  [KP_PID_distance] -> Divide/1
  Delay4/1 -> Add4/2
  Add3/1 -> Divide1/1, Gain/1
  Divide2/1 -> Add2/3
  Divide/1 -> Add2/1
  err/1 -> Add4/1, Add3/1, Divide/2, Delay4/1
  [KD_PID_distance] -> Divide2/2

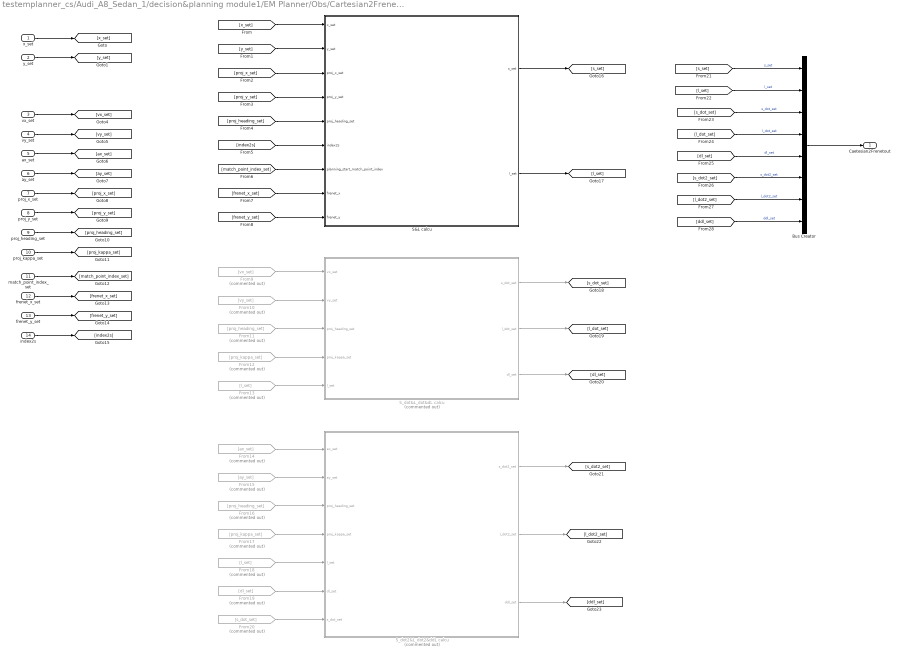
== system testemplanner_cs/Audi_A8_Sedan_1/decision&planning module1/EM Planner/Obs/Cartesian2Frenet-static obs ==
  x_set : Inport
  y_set : Inport  Port=2
  vx_set : Inport  Port=3
  vy_set : Inport  Port=4
  ax_set : Inport  Port=5
  ay_set : Inport  Port=6
  proj_x_set : Inport  Port=7
  proj_y_set : Inport  Port=8
  proj_heading_set : Inport  Port=9
  proj_kappa_set : Inport  Port=10
  match_point_index_set : Inport  Port=11
  frenet_x_set : Inport  Port=12
  frenet_y_set : Inport  Port=13
  index2s : Inport  Port=14
  Bus Creator : BusCreator  Inputs=8
  From10 : From  Commented=on  GotoTag=vy_set
  From11 : From  Commented=on  GotoTag=proj_heading_set
  From12 : From  Commented=on  GotoTag=proj_kappa_set
  From13 : From  Commented=on  GotoTag=l_set
  From14 : From  Commented=on  GotoTag=ax_set
  From15 : From  Commented=on  GotoTag=ay_set
  From16 : From  Commented=on  GotoTag=proj_heading_set
  From17 : From  Commented=on  GotoTag=proj_kappa_set
  From18 : From  Commented=on  GotoTag=l_set
  From19 : From  Commented=on  GotoTag=dl_set
  From20 : From  Commented=on  GotoTag=s_dot_set
  From9 : From  Commented=on  GotoTag=vx_set
  S&L calcu : MATLAB Function  TreatAsAtomicUnit=on
  "S_dot&L_dot&dL calcu " : MATLAB Function  Commented=on  TreatAsAtomicUnit=on
  S_dot2&L_dot2&ddL calcu : MATLAB Function  Commented=on  TreatAsAtomicUnit=on
  Caetesian2Frenetout : Outport
  wires:
  Bus Creator/1 -> Caetesian2Frenetout/1
  [ddl_set] -> Bus Creator/8  "ddl_set"
  [l_dot2_set] -> Bus Creator/7  "l_dot2_set"
  [s_dot2_set] -> Bus Creator/6  "s_dot2_set"
  [dl_set] -> Bus Creator/5  "dl_set"
  [l_dot_set] -> Bus Creator/4  "l_dot_set"
  [s_dot_set] -> Bus Creator/3  "s_dot_set"
  [l_set] -> Bus Creator/2  "l_set"
  [s_set] -> Bus Creator/1  "s_set"
  S_dot2&L_dot2&ddL calcu/3(ddl_set) -> [ddl_set]
  S_dot2&L_dot2&ddL calcu/2(l_dot2_set) -> [l_dot2_set]
  S_dot2&L_dot2&ddL calcu/1(s_dot2_set) -> [s_dot2_set]
  From20/1 -> S_dot2&L_dot2&ddL calcu/7(s_dot_set)
  From19/1 -> S_dot2&L_dot2&ddL calcu/6(dl_set)
  From18/1 -> S_dot2&L_dot2&ddL calcu/5(l_set)
  From17/1 -> S_dot2&L_dot2&ddL calcu/4(proj_kappa_set)
  From16/1 -> S_dot2&L_dot2&ddL calcu/3(proj_heading_set)
  From15/1 -> S_dot2&L_dot2&ddL calcu/2(ay_set)
  From14/1 -> S_dot2&L_dot2&ddL calcu/1(ax_set)
  "S_dot&L_dot&dL calcu "/3(dl_set) -> [dl_set]
  "S_dot&L_dot&dL calcu "/2(l_dot_set) -> [l_dot_set]
  "S_dot&L_dot&dL calcu "/1(s_dot_set) -> [s_dot_set]
  From13/1 -> "S_dot&L_dot&dL calcu "/5(l_set)
  S&L calcu/2(l_set) -> [l_set]
  S&L calcu/1(s_set) -> [s_set]
  From12/1 -> "S_dot&L_dot&dL calcu "/4(proj_kappa_set)
  From11/1 -> "S_dot&L_dot&dL calcu "/3(proj_heading_set)
  From10/1 -> "S_dot&L_dot&dL calcu "/2(vy_set)
  From9/1 -> "S_dot&L_dot&dL calcu "/1(vx_set)
  [frenet_y_set] -> S&L calcu/9(frenet_y)
  [frenet_x_set] -> S&L calcu/8(frenet_x)
  [match_point_index_set] -> S&L calcu/7(planning_start_match_point_index)
  [index2s] -> S&L calcu/6(index2s)
  [proj_heading_set] -> S&L calcu/5(proj_heading_set)
  [x_set] -> S&L calcu/1(x_set)
  [proj_y_set] -> S&L calcu/4(proj_y_set)
  [proj_x_set] -> S&L calcu/3(proj_x_set)
  [y_set] -> S&L calcu/2(y_set)
  index2s/1 -> [index2s]
  frenet_y_set/1 -> [frenet_y_set]
  frenet_x_set/1 -> [frenet_x_set]
  match_point_index_set/1 -> [match_point_index_set]
  proj_kappa_set/1 -> [proj_kappa_set]
  proj_heading_set/1 -> [proj_heading_set]
  proj_y_set/1 -> [proj_y_set]
  proj_x_set/1 -> [proj_x_set]
  ay_set/1 -> [ay_set]
  ax_set/1 -> [ax_set]
  vy_set/1 -> [vy_set]
  vx_set/1 -> [vx_set]
  y_set/1 -> [y_set]
  x_set/1 -> [x_set]

== matlab function testemplanner_cs/Audi_A8_Sedan_1/control module/control main/lateral control LQR/feed_forword_control ==
  data: vx input; a input; forword_angle output; b input; m input; cf input; cr input; k input; kr input
function forword_angle = fcn(vx,a,b,m,cf,cr,k,kr)
    forword_angle=kr*(a+b-b*k(3)-(m*vx*vx/(a+b))*((b/cf)+(a/cr)*k(3)-(a/cr)));
end

== matlab function testemplanner_cs/Audi_A8_Sedan_1/control module/control main/lateral control LQR/feedback_control+feedforword_control ==
  data: k input; angle output; err input; forword_angle input
function angle = fcn(k,err,forword_angle)

    angle=-k*err+forword_angle;
end

== matlab function testemplanner_cs/Audi_A8_Sedan_1/control module/control main/lateral control LQR/calc lqr K ==
  data: k1 input; k output; k2 input; k3 input; k4 input; vx input
function k  = fcn(k1,k2,k3,k4,vx)
    if abs(vx)<0.1
        k=[0,0,0,0];
    else
       
        k=[k1,k2,k3,k4];
    end
end

== matlab function testemplanner_cs/Audi_A8_Sedan_1/control module/control main/lateral control LQR/predict_module ==
  data: x input; pred_x_ctrl output; y input; phi input; vx input; vy input; phi_dot input; ts input; pred_y_ctrl output; pred_yaw_ctrl output; pred_vx_ctrl output; pred_vy_ctrl output; pred_yaw_dot_ctrl output
function [pred_x_ctrl,pred_y_ctrl,pred_yaw_ctrl,pred_vx_ctrl,pred_vy_ctrl,pred_yaw_dot_ctrl] = fcn(x,y,phi,vx,vy,phi_dot,ts)
    pred_x_ctrl=x+vx*ts*cos(phi)-vy*ts*sin(phi);
    pred_y_ctrl=y+vy*ts*cos(phi)+vx*ts*sin(phi);
    pred_yaw_ctrl=phi;
    pred_vx_ctrl=vx;
    pred_vy_ctrl=vy;
    pred_yaw_dot_ctrl=phi_dot;
end

== matlab function testemplanner_cs/Audi_A8_Sedan_1/decision&planning module1/EM Planner/Cartesian2Frenet-panning start point/S&L calcu ==
  data: s_set output; l_set output; x_set input; y_set input; proj_x_set input; proj_y_set input; proj_heading_set input; index2s input; planning_start_match_point_index input; frenet_x input; frenet_y input
function [s_set, l_set] = fcn(x_set, y_set, proj_x_set, proj_y_set, proj_heading_set, index2s, ...
    planning_start_match_point_index, frenet_x, frenet_y)

%此函数用来存储规划起点及障碍物在以自车定位的投影点为参考线原点的frenet坐标系的sl坐标
%由于不知道规划起点及障碍物共多少个，故需要缓冲
%计算s时直接复用index2s模块中写好的子函数
%共有128个点

n = 128;
s_set = ones(n,1)*nan;
l_set = ones(n,1)*nan;
 
for i = 1:length(x_set)
    if isnan(x_set(i))
        break;
    end
    %计算规划起点或障碍物的匹配点到参考线原点(自车在参考线上的投影点)的弧长
    s_set(i) = CalcSFromIndex2s(index2s, planning_start_match_point_index, proj_x_set(i), proj_y_set(i), frenet_x, frenet_y);
    vector_rh = [x_set(i); y_set(i)];
    vector_rr = [proj_x_set(i); proj_y_set(i)];
    vector_nor_r = [-sin(proj_heading_set(i)); cos(proj_heading_set(i))];
    l_set(i) = (vector_rh-vector_rr)'*vector_nor_r;
end
end

%复用index2s中写好的计算弧长s的子函数
function s0 = CalcSFromIndex2s(index2s, match_point_index, proj_x, proj_y, path_x, path_y)
%该函数第一次调用时用来计算自车投影点到参考线起点的弧长！！！
%该函数复用时用来计算障碍物投影点到参考线原点的弧长！！！
%我认为这里第一次使用与复用时的逻辑混乱，非常复杂

%我们要计算参考线起点到投影点（坐标系原点）的弧长
%并且已知参考线起点到匹配点的弧长index2s（i）
%所以要计算投影点与匹配点间的距离和相对位置关系
%向量的内积可以判断位置关系

%先定义投影点与匹配点的误差向量
vector1 = [proj_x; proj_y]-[path_x(match_point_index); path_y(match_point_index)];

%可以根据匹配点的临近点近似描述匹配点的方向向量
%1：如果匹配点前面还有点
%2：如果匹配点是最后一个点
if match_point_index < length(path_x)
    %定义匹配点的切向量
    vector2 = [path_x(match_point_index+1)-path_x(match_point_index); path_y(match_point_index+1)-path_y(match_point_index)];
else
    vector2 = [path_x(match_point_index)-path_x(match_point_index-1); path_y(match_point_index)-path_y(match_point_index-1)];
end

%判断匹配点与投影点的相对位置关系
%计算参考线起点到投影点的弧长
if vector1'*vector2 > 0
    %投影点在前，匹配点在后
    s0 = index2s(match_point_index)+sqrt(vector1'*vector1);
else
    %匹配点在前，投影点在后
    s0 = index2s(match_point_index)-sqrt(vector1'*vector1);
end
end

== matlab function testemplanner_cs/Audi_A8_Sedan_1/control module/MATLAB Function ==
  data: current_time input; xr output; trajectory_x input; trajectory_y input; trajectory_heading input; trajectory_kappa input; trajectory_speed input; trajectory_accel input; yr output; thetar output; kappar output; speedr output; accelr output; trajectory_time input
function [xr, yr, thetar, kappar, speedr, accelr] = fcn(current_time, trajectory_x, trajectory_y, trajectory_heading...
    , trajectory_kappa, trajectory_speed, trajectory_accel, trajectory_time)

%因为控制接受的信号不再是一个点，而是一个序列，因此要找出控制时间对应的轨迹信息
%控制也有延迟，因此控制跟踪的点的时间应该是当前时间+10ms

control_time = current_time+0.01;

%由于轨迹是拼接而成的，若无拼接轨迹，stitch_time中的信息应该是-1
%所以要找到时间信息中第一个不是-1的点
index = 1;
while trajectory_time(index) == -1
    index = index+1;
end

%用inerp1对时间插值，simulink中该函数要求自变量是线性变化的，且插值时间应该在插值范围之内
%若待插点处在范围边界或之外，会发生报错
%规划的周期是100ms,意味着第一次规划还未完成控制已经执行了十次
%控制跟踪的是一条空轨迹：0,0,0,0,0...,trajectory_time也全部为0(非线性)
%上述情况只可能发生在仿真刚开始时
if control_time > trajectory_time(index) && trajectory_time(index) ~= 0
    xr = interp1(trajectory_time(index:end), trajectory_x(index:end), control_time);
    yr = interp1(trajectory_time(index:end), trajectory_y(index:end), control_time);
    thetar = interp1(trajectory_time(index:end), trajectory_heading(index:end), control_time);
    kappar = interp1(trajectory_time(index:end), trajectory_kappa(index:end), control_time);
    speedr = interp1(trajectory_time(index:end), trajectory_speed(index:end), control_time);
    accelr = interp1(trajectory_time(index:end), trajectory_accel(index:end), control_time);
else
    xr = trajectory_x(index);
    yr = trajectory_y(index);
    thetar = trajectory_heading(index);
    kappar = trajectory_kappa(index);
    speedr = trajectory_speed(index);
    accelr = trajectory_accel(index);
end

== matlab function testemplanner_cs/Audi_A8_Sedan_1/decision&planning module1/EM Planner/Cartesian2Frenet-panning start point/S_dot&L_dot&dL calcu  ==
  data: s_dot_set output; vx_set input; vy_set input; proj_heading_set input; proj_kappa_set input; l_set input; l_dot_set output; dl_set output
function [s_dot_set, l_dot_set, dl_set]  = fcn(vx_set, vy_set, proj_heading_set, proj_kappa_set, l_set)

%这个函数用来存储s_dot&l_dot&dl的集合
n = 128;
s_dot_set = ones(n,1)*nan;
l_dot_set = ones(n,1)*nan;
dl_set = ones(n,1)*nan;

for i = 1:length(l_set)
    if isnan(l_set(i))
        break;
    end
    vector_vh = [vx_set(i); vy_set(i)];
    vector_tor_r = [cos(proj_heading_set(i)); sin(proj_heading_set(i))];
    vector_nor_r = [-sin(proj_heading_set(i)); cos(proj_heading_set(i))];
    s_dot_set(i) = vector_vh'*vector_tor_r/(1-proj_kappa_set(i)*l_set(i));
    l_dot_set(i) = vector_vh'*vector_nor_r;

    %dl=l_dot/s_dot,所以s_dot不能为0，这里要打一个补丁，当s_dot趋于0时，dl=0
    if abs(s_dot_set(i)) < 1e-6
        dl_set(i) = 0;
    else
        dl_set(i) = l_dot_set(i)/s_dot_set(i);
    end

end

end

== matlab function testemplanner_cs/Audi_A8_Sedan_1/decision&planning module1/EM Planner/Cartesian2Frenet-panning start point/S_dot2&L_dot2&ddL calcu ==
  data: ax_set input; s_dot2_set output; ay_set input; proj_heading_set input; proj_kappa_set input; l_set input; dl_set input; s_dot_set input; l_dot2_set output; ddl_set output
function [s_dot2_set, l_dot2_set, ddl_set] = fcn(ax_set, ay_set, proj_heading_set, proj_kappa_set, l_set, dl_set...
    , s_dot_set)

%该函数用来存储s_dot2&l_dot2&ddl,同样要设置缓冲
n = 128;
s_dot2_set = ones(n,1)*nan;
l_dot2_set = ones(n,1)*nan; 
ddl_set = ones(n,1)*nan;

for i = 1:length(l_set)
    if isnan(l_set(i))
        break;
    end
    vector_ah = [ax_set(i); ay_set(i)];
    vector_tor_r = [cos(proj_heading_set(i)); sin(proj_heading_set(i))];
    vector_nor_r = [-sin(proj_heading_set(i)); cos(proj_heading_set(i))];

    %kr'=dkr/ds,曲率随弧长的变化速率很小，kr'=0
    s_dot2_set(i) = vector_ah'*vector_tor_r/(1-proj_kappa_set(i)*l_set(i))+proj_kappa_set(i)*dl_set(i)*s_dot_set(i)^2/(1-proj_kappa_set(i)*l_set(i))...
        +s_dot_set(i)^2*proj_kappa_set(i)*dl_set(i)/(1-proj_kappa_set(i)*l_set(i));

    l_dot2_set(i) = vector_ah'*vector_nor_r-proj_kappa_set(i)*s_dot_set(i)^2*(1-proj_kappa_set(i)*l_set(i));

    %ddl的表达式分母上有s_dot,同样要确保s_dot不为0
    if abs(s_dot_set(i)) < 1e-6
        ddl_set(i) = 0;
    else
        ddl_set(i) = (l_dot2_set(i)-dl_set(i)*s_dot2_set(i))/s_dot_set(i)^2; 
    end

end

end
